simulink model "Controller_Deliverable_1"  (R2024a)
settings: Solver=VariableStepAuto  StartTime=0.0  StopTime=inf  RelTol=1e-3
libraries: robotlib x5
settings Model: Creator=carlosortiz  LastModifiedBy=suryachand

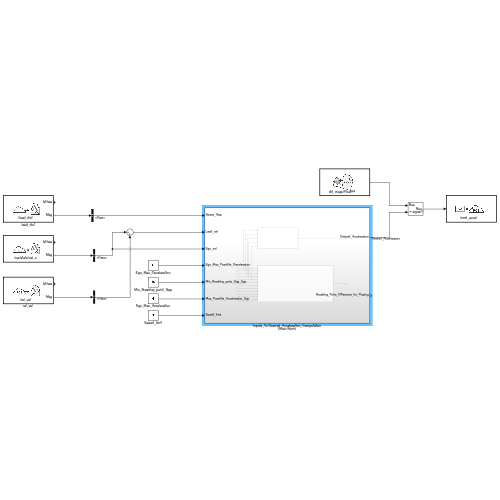
[thumbnail: Simulink's stored preview of the top-level diagram]
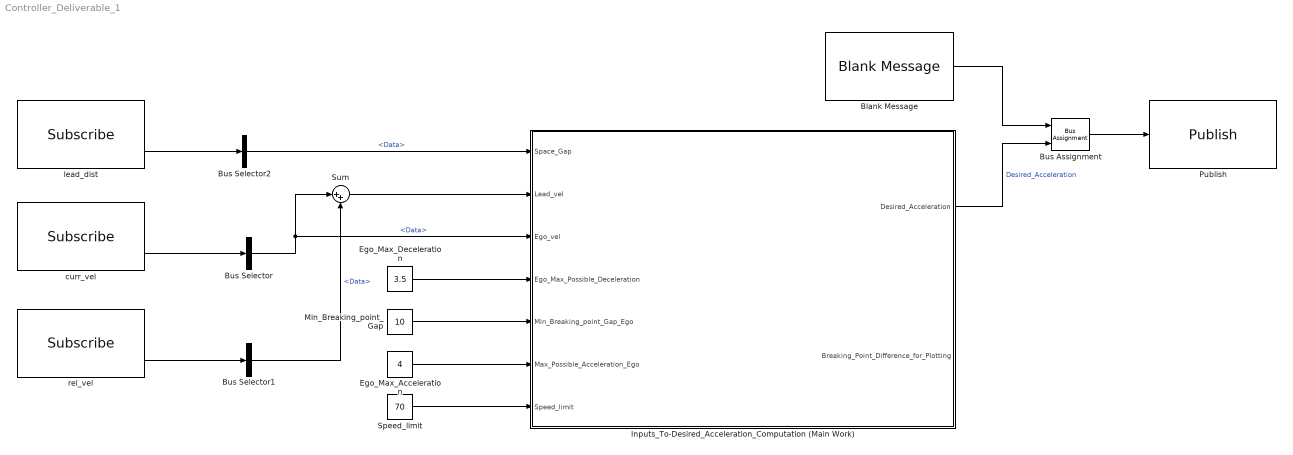
== system Controller_Deliverable_1 ==
  Blank Message : robotlib/Blank Message  messageClass=Message  entityType=std_msgs/Float64  messageType=std_msgs/Float64  SampleTime=inf  legacyBusStruct=off
  Bus Assignment : BusAssignment  AssignedSignals=signal1
  Bus Selector : BusSelector  OutputSignals=Data
  Bus Selector1 : BusSelector  OutputSignals=Data
  Bus Selector2 : BusSelector  OutputSignals=Data
  Ego_Max_Acceleration : Constant  Value=4
  Ego_Max_Deceleration : Constant  Value=3.5
  Inputs_To-Desired_Acceleration_Computation (Main Work) : Subsystem
  Min_Breaking_point_Gap : Constant  Value=10
  Publish : robotlib/Publish  topicSource=Specify your own  topic=/cmd_accel  messageType=std_msgs/Float64  legacyBusStruct=off  messageQueueLength=1
  Speed_limit : Constant  Value=70
  Sum : Sum  Inputs=|++
  curr_vel : robotlib/Subscribe  topicSource=Specify your own  topic=/car/state/vel_x  messageType=std_msgs/Float64  SampleTime=-1  legacyBusStruct=off  messageQueueLength=1
  lead_dist : robotlib/Subscribe  topicSource=Specify your own  topic=/lead_dist  messageType=std_msgs/Float64  SampleTime=-1  legacyBusStruct=off  messageQueueLength=1
  rel_vel : robotlib/Subscribe  topicSource=Specify your own  topic=/rel_vel  messageType=std_msgs/Float64  SampleTime=-1  legacyBusStruct=off  messageQueueLength=1
  wires:
  curr_vel/2 -> Bus Selector/1
  rel_vel/2 -> Bus Selector1/1
  lead_dist/2 -> Bus Selector2/1
  Bus Selector2/1 -> Inputs_To-Desired_Acceleration_Computation (Main Work)/1(Space_Gap)  "<Data>"
  Bus Selector/1 -> Sum/1, Inputs_To-Desired_Acceleration_Computation (Main Work)/3(Ego_vel)  "<Data>"
  Sum/1 -> Inputs_To-Desired_Acceleration_Computation (Main Work)/2(Lead_vel)
  Bus Selector1/1 -> Sum/2  "<Data>"
  Blank Message/1 -> Bus Assignment/1
  Inputs_To-Desired_Acceleration_Computation (Main Work)/1(Desired_Acceleration) -> Bus Assignment/2  "Desired_Acceleration"
  Bus Assignment/1 -> Publish/1
  Ego_Max_Deceleration/1 -> Inputs_To-Desired_Acceleration_Computation (Main Work)/4(Ego_Max_Possible_Deceleration)
  Min_Breaking_point_Gap/1 -> Inputs_To-Desired_Acceleration_Computation (Main Work)/5(Min_Breaking_point_Gap_Ego)
  Ego_Max_Acceleration/1 -> Inputs_To-Desired_Acceleration_Computation (Main Work)/6(Max_Possible_Acceleration_Ego)
  Speed_limit/1 -> Inputs_To-Desired_Acceleration_Computation (Main Work)/7(Speed_limit)

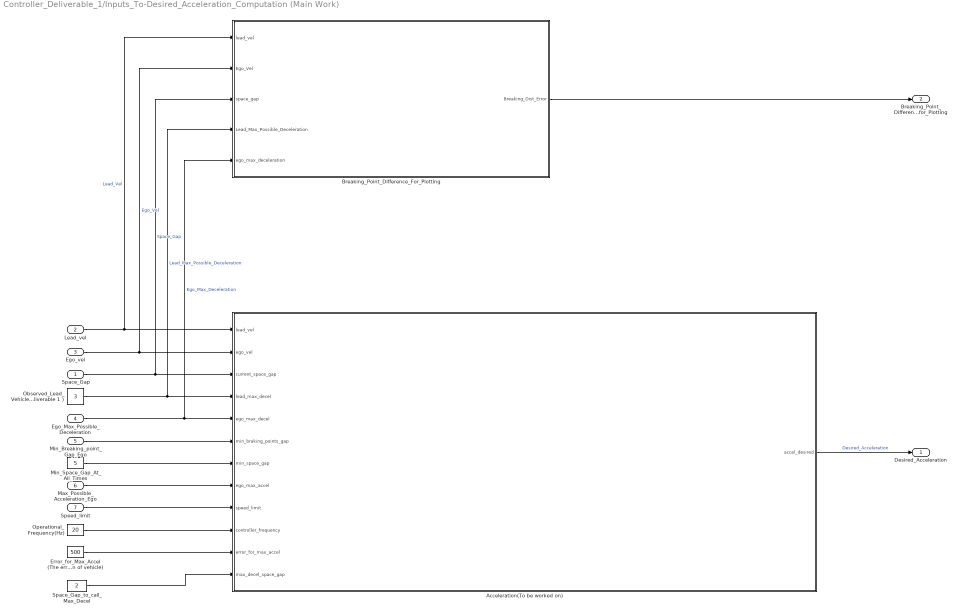
== system Controller_Deliverable_1/Inputs_To-Desired_Acceleration_Computation (Main Work) ==
  Space_Gap : Inport
  Lead_vel : Inport  Port=2
  Ego_vel : Inport  Port=3
  Ego_Max_Possible_Deceleration : Inport  Port=4
  Min_Breaking_point_Gap_Ego : Inport  Port=5
  Max_Possible_Acceleration_Ego : Inport  Port=6
  Speed_limit : Inport  Port=7
  Acceleration(To be worked on) : MATLAB Function  TreatAsAtomicUnit=on
  Breaking_Point_Difference_For_Plotting : Subsystem
  Error_for_Max_Accel (The error distance in breaking points which is threshold for using max acceleration of vehicle) : Constant  Value=500
  Min_Space_Gap_At_All_Times : Constant  Value=5
  Observed_Lead_Vehicle_Max_Deceleration (For now keeping one fixed value to all vehicles for scope of deliverable 1 ) : Constant  Value=3
  Operational_Frequency(Hz) : Constant  Value=20
  Space_Gap_to_call_Max_Decel : Constant  Value=2
  Desired_Acceleration : Outport
  Breaking_Point_Difference_for_Plotting : Outport  Port=2
  wires:
  Acceleration(To be worked on)/1(accel_desired) -> Desired_Acceleration/1  "Desired_Acceleration"
  Min_Breaking_point_Gap_Ego/1 -> Acceleration(To be worked on)/6(min_braking_points_gap)
  Max_Possible_Acceleration_Ego/1 -> Acceleration(To be worked on)/8(ego_max_accel)
  Speed_limit/1 -> Acceleration(To be worked on)/9(speed_limit)
  Min_Space_Gap_At_All_Times/1 -> Acceleration(To be worked on)/7(min_space_gap)
  Operational_Frequency(Hz)/1 -> Acceleration(To be worked on)/10(controller_frequency)
  Error_for_Max_Accel (The error distance in breaking points which is threshold for using max acceleration of vehicle)/1 -> Acceleration(To be worked on)/11(error_for_max_accel)
  Space_Gap_to_call_Max_Decel/1 -> Acceleration(To be worked on)/12(max_decel_space_gap)
  Space_Gap/1 -> Acceleration(To be worked on)/3(current_space_gap), Breaking_Point_Difference_For_Plotting/3(space_gap)  "Space_Gap"
  Ego_Max_Possible_Deceleration/1 -> Acceleration(To be worked on)/5(ego_max_decel), Breaking_Point_Difference_For_Plotting/5(ego_max_deceleration)  "Ego_Max_Deceleration"
  Observed_Lead_Vehicle_Max_Deceleration (For now keeping one fixed value to all vehicles for scope of deliverable 1 )/1 -> Acceleration(To be worked on)/4(lead_max_decel), Breaking_Point_Difference_For_Plotting/4(Lead_Max_Possible_Deceleration)  "Lead_Max_Possible_Deceleration"
  Ego_vel/1 -> Acceleration(To be worked on)/2(ego_vel), Breaking_Point_Difference_For_Plotting/2(Ego_Vel)  "Ego_Vel"
  Lead_vel/1 -> Acceleration(To be worked on)/1(lead_vel), Breaking_Point_Difference_For_Plotting/1(lead_vel)  "Lead_Vel"
  Breaking_Point_Difference_For_Plotting/1(Breaking_Dist_Error) -> Breaking_Point_Difference_for_Plotting/1

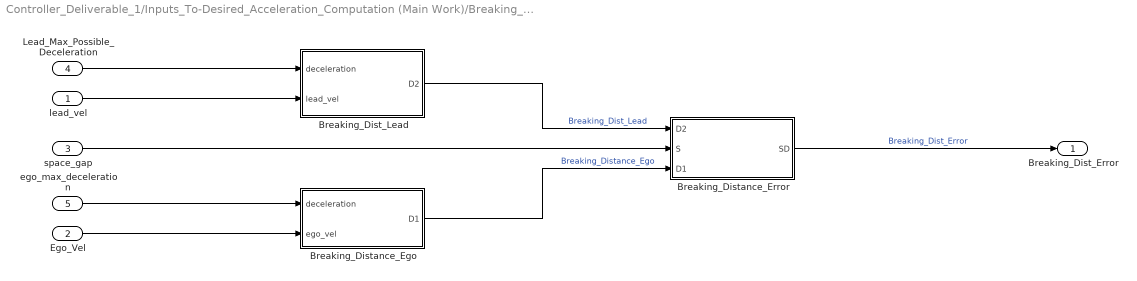
== system Controller_Deliverable_1/Inputs_To-Desired_Acceleration_Computation (Main Work)/Breaking_Point_Difference_For_Plotting ==
  lead_vel : Inport
  Ego_Vel : Inport  Port=2
  space_gap : Inport  Port=3
  Lead_Max_Possible_Deceleration : Inport  Port=4
  ego_max_deceleration : Inport  Port=5
  Breaking_Dist_Lead : MATLAB Function  TreatAsAtomicUnit=on
  Breaking_Distance_Ego : MATLAB Function  TreatAsAtomicUnit=on
  Breaking_Distance_Error : MATLAB Function  TreatAsAtomicUnit=on
  Breaking_Dist_Error : Outport
  wires:
  Ego_Vel/1 -> Breaking_Distance_Ego/2(ego_vel)
  space_gap/1 -> Breaking_Distance_Error/2(S)
  lead_vel/1 -> Breaking_Dist_Lead/2(lead_vel)
  ego_max_deceleration/1 -> Breaking_Distance_Ego/1(deceleration)
  Breaking_Distance_Error/1(SD) -> Breaking_Dist_Error/1  "Breaking_Dist_Error"
  Breaking_Distance_Ego/1(D1) -> Breaking_Distance_Error/3(D1)  "Breaking_Distance_Ego"
  Lead_Max_Possible_Deceleration/1 -> Breaking_Dist_Lead/1(deceleration)
  Breaking_Dist_Lead/1(D2) -> Breaking_Distance_Error/1(D2)  "Breaking_Dist_Lead"

== matlab function Controller_Deliverable_1/Inputs_To-Desired_Acceleration_Computation (Main Work)/Acceleration(To be worked on) ==
  data: accel_desired output; lead_vel input; ego_vel input; current_space_gap input; lead_max_decel input; ego_max_decel input; min_braking_points_gap input; min_space_gap input; ego_max_accel input; speed_limit input; controller_frequency input; error_for_max_accel input; max_decel_space_gap input
function accel_desired = accel_ctrl_(lead_vel, ego_vel, current_space_gap, ...
    lead_max_decel, ego_max_decel, min_braking_points_gap, min_space_gap, ...
    ego_max_accel, speed_limit, controller_frequency, error_for_max_accel, max_decel_space_gap)
    % ACCEL_CTRL_ Calculates the desired acceleration for the ego vehicle to maintain
    % a safe following distance behind a lead vehicle while considering vehicle capabilities
    % and safety constraints.
    %
    % Parameters:
    %   lead_vel                - Velocity of the lead vehicle (m/s)
    %   ego_vel                 - Current velocity of the ego vehicle (m/s)
    %   current_space_gap       - Current distance between ego and lead vehicles (m)
    %   lead_max_decel          - Maximum deceleration capability of the lead vehicle (m/s²)
    %   ego_max_decel           - Maximum deceleration capability of the ego vehicle (m/s²)
    %   min_braking_points_gap  - Minimum desired gap based on braking points (m)
    %   min_space_gap           - Absolute minimum safe space gap (m)
    %   ego_max_accel           - Maximum acceleration capability of the ego vehicle (m/s²)
    %   speed_limit             - Speed limit of the road (m/s) [Not used in current implementation]
    %   controller_frequency    - Frequency at which the controller operates (Hz)
    %   error_for_max_accel     - Error threshold at which maximum acceleration is applied (m)
    %   max_decel_space_gap     - Additional space gap for maximum deceleration (m)
    %
    % Returns:
    %   accel_desired - The desired acceleration command for the ego vehicle (m/s²)
    
    % Constants
    f = 0.55; % Coefficient of friction between tires and road
    g = 9.8;  % Acceleration due to gravity (m/s²)

    % Time step calculation based on controller frequency
    dt = 1 / controller_frequency;

    % Step 1: Initialize Working Variables
    % -------------------------------------
    % These variables may be adjusted based on the relative deceleration capabilities
    % of the ego and lead vehicles.
    working_decel_ego = ego_max_decel;   % Working maximum deceleration of ego vehicle
    working_decel_lead = lead_max_decel; % Working maximum deceleration of lead vehicle
    working_min_gap = min_braking_points_gap; % Minimum braking point gap

    % Conditional Adjustment Based on Maximum Decelerations
    if ego_max_decel > lead_max_decel
        % If ego vehicle can decelerate faster than lead vehicle,
        % limit ego's deceleration to lead's maximum deceleration to maintain safety.
        working_decel_ego = lead_max_decel;

        % Adjust the working minimum gap to ensure safety
        working_min_gap = min(min_space_gap, min_braking_points_gap);
    end

    % Step 2: Calculate Stopping Distances
    % -------------------------------------
    % Calculate the stopping distances for both ego and lead vehicles.
    % The stopping distance accounts for both the distance required to stop and
    % the distance covered due to friction.
    D1 = (ego_vel^2 / (2 * working_decel_ego)) + ((ego_vel^2 / (2 * g)) * f);
    D2 = (lead_vel^2 / (2 * working_decel_lead)) + ((lead_vel^2 / (2 * g)) * f);

    % Step 3: Compute the Stopping Distance Error
    % -------------------------------------------
    % Determine how much the current stopping distance deviates from the desired minimum gap.
    stop_dist = (D2 + current_space_gap) - D1;
    error = stop_dist - working_min_gap;

    % Step 4: Map Error to Desired Acceleration Using Different Gamma Values
    % ------------------------------------------------------------------------
    % Depending on whether the error indicates a need to accelerate or decelerate,
    % apply different responsiveness levels using gamma values.
    % gamma_neg controls responsiveness during deceleration.
    % gamma_pos controls responsiveness during acceleration.
    gamma_neg = 1; % For deceleration (negative errors)
    gamma_pos = 2; % For acceleration (positive errors)

    % Define Thresholds for Applying Maximum Acceleration or Deceleration
    threshold_decel_error = -(working_min_gap - max_decel_space_gap); % Negative threshold
    threshold_accel_error = error_for_max_accel; % Positive threshold

    if error >= threshold_accel_error
        % Case 1: Error exceeds the positive threshold
        % Apply maximum acceleration.
        accel_desired = ego_max_accel;
    elseif error >= 0
        % Case 2: Error is positive but below the threshold
        % Apply a non-linear (quadratic) mapping to determine desired acceleration.
        accel_desired = ego_max_accel * (error / threshold_accel_error)^gamma_pos;
    elseif error <= threshold_decel_error
        % Case 3: Error exceeds the negative threshold
        % Apply maximum deceleration.
        accel_desired = -ego_max_decel;
    else
        % Case 4: Error is negative but above the threshold
        % Apply a non-linear (linear in this case) mapping to determine desired deceleration.
        % The fraction (error / threshold_decel_error) is positive.
        accel_desired = -ego_max_decel * (error / threshold_decel_error)^gamma_neg;
    end

    % Step 5: One-Step Lookahead
    % ---------------------------
    % Predict the future positions of both ego and lead vehicles after one time step (dt)
    % to ensure that the desired acceleration maintains a safe following distance.
    
    % Predict Future Position of Ego Vehicle
    % Using the kinematic equation: s = ut + 0.5 * a * t²
    ego_future_pos = ego_vel * dt + 0.5 * accel_desired * dt^2; % Assuming current position is 0

    % Predict Future Position of Lead Vehicle
    % Assuming the lead vehicle maintains constant velocity.
    lead_future_pos = current_space_gap + lead_vel * dt;

    % Compute Future Space Gap Between Lead and Ego Vehicles
    future_space_gap = lead_future_pos - ego_future_pos;

    % Adjust Desired Acceleration if Future Space Gap is Less Than Minimum Safe Gap
    if future_space_gap < min_space_gap
        % Calculate the required acceleration to maintain the minimum space gap.
        delta_s = (current_space_gap + lead_vel * dt) - (ego_vel * dt + min_space_gap);
        accel_required = (2 * (delta_s - ego_vel * dt)) / dt^2;

        % Adjust accel_desired to prevent collision by choosing the smaller acceleration.
        accel_desired = min(accel_required, accel_desired);

        % Ensure accel_desired remains within the vehicle's acceleration limits.
        accel_desired = min(accel_desired, ego_max_accel);
        accel_desired = max(accel_desired, -ego_max_decel);
    end

    % Step 6: Final Clipping of Desired Acceleration
    % -----------------------------------------------
    % Ensure that the calculated desired acceleration does not exceed the vehicle's
    % physical capabilities by clipping it within the allowable range.
    accel_desired = min(accel_desired, ego_max_accel);    % Limit to maximum acceleration
    accel_desired = max(accel_desired, -ego_max_decel);   % Limit to maximum deceleration
end

== matlab function Controller_Deliverable_1/Inputs_To-Desired_Acceleration_Computation (Main Work)/Breaking_Point_Difference_For_Plotting/Breaking_Distance_Error ==
  data: D2 input; SD output; S input; D1 input
function SD = stop_dist_diff(D2, S, D1)

SD = (D2+S)-D1;

== matlab function Controller_Deliverable_1/Inputs_To-Desired_Acceleration_Computation (Main Work)/Breaking_Point_Difference_For_Plotting/Breaking_Distance_Ego ==
  data: deceleration input; D1 output; ego_vel input
function D1 = D1(deceleration, ego_vel)
    f=0.55; % coeff. friction
    g=9.8;
    D1 = (ego_vel^2 / (2*deceleration))+((ego_vel^2/(2*g))*f);

== matlab function Controller_Deliverable_1/Inputs_To-Desired_Acceleration_Computation (Main Work)/Breaking_Point_Difference_For_Plotting/Breaking_Dist_Lead ==
  data: deceleration input; lead_vel input; D2 output
function D2 = D2(deceleration, lead_vel)
    f=0.55; % coeff. friction
    g=9.8;
    D2 = (lead_vel^2 / (2*deceleration))+((lead_vel^2/(2*g))*f);
